simulink model "TST_DYN"  (R2020a)
settings: Solver=FixedStepAuto  StartTime=0.0  StopTime=10000  FixedStep=1  RelTol=1e-3
libraries: DYN x1
settings Model: Creator=WilTravis  LastModifiedBy=m_mam
settings DataIOCC: ReturnWorkspaceOutputs=off
settings DebuggingCC: ArithmeticOperatorsInVariantConditions=warning
settings SFSimCC: SimUseLocalCustomCode=off  CustomCodeUndefinedFunction=UseInterfaceOnly
settings RTWCC: RTWUseLocalCustomCode=off

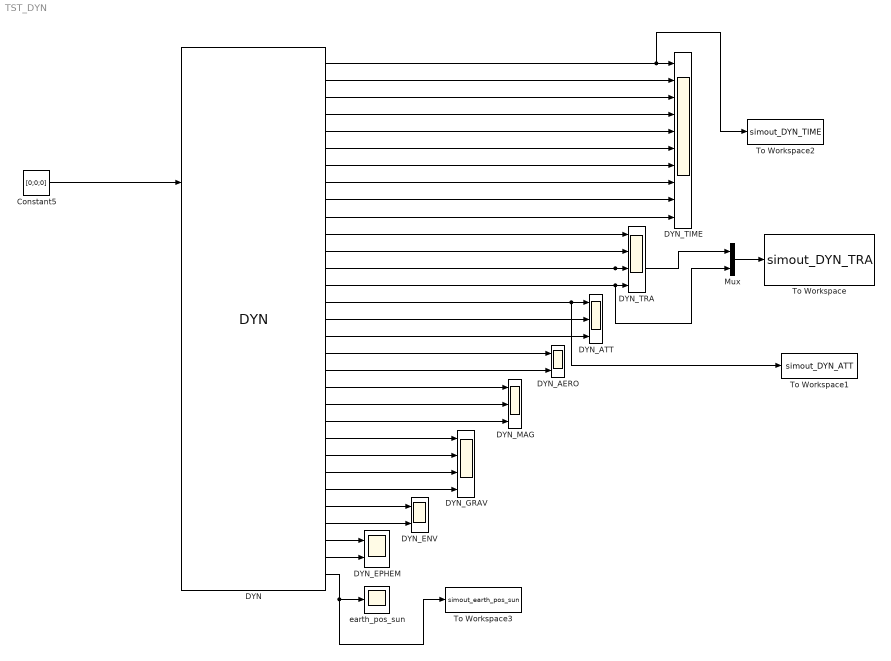
== system TST_DYN ==
  Constant5 : Constant  Value=[0;0;0]
  DYN : DYN/DYN  SystemSampleTime=-1  Latency=0  AutoFrameSizeCalculation=off
  DYN_AERO : Scope  NumInputPorts=2
  DYN_ATT : Scope  NumInputPorts=3
  DYN_ENV : Scope  NumInputPorts=2
  DYN_EPHEM : Scope  NumInputPorts=2
  DYN_GRAV : Scope  NumInputPorts=4
  DYN_MAG : Scope  NumInputPorts=3
  DYN_TIME : Scope  NumInputPorts=10
  DYN_TRA : Scope  NumInputPorts=4
  Mux : Mux  Inputs=2
  To Workspace : ToWorkspace  VariableName=simout_DYN_TRA  SaveFormat=Timeseries  SampleTime=-1
  To Workspace1 : ToWorkspace  VariableName=simout_DYN_ATT  SaveFormat=Timeseries  SampleTime=-1
  To Workspace2 : ToWorkspace  VariableName=simout_DYN_TIME  SaveFormat=Timeseries  SampleTime=-1
  To Workspace3 : ToWorkspace  VariableName=simout_earth_pos_sun  SaveFormat=Timeseries  SampleTime=-1
  earth_pos_sun : Scope
  wires:
  Constant5/1 -> DYN/1
  DYN/20 -> DYN_MAG/1
  DYN/12 -> DYN_TRA/2
  DYN/2 -> DYN_TIME/2
  DYN/28 -> DYN_ENV/2
  DYN/6 -> DYN_TIME/6
  DYN/23 -> DYN_GRAV/1
  DYN/13 -> Mux/1, DYN_TRA/3
  DYN/11 -> DYN_TRA/1
  DYN/15 -> DYN_ATT/1, To Workspace1/1
  DYN/19 -> DYN_AERO/2
  DYN/3 -> DYN_TIME/3
  DYN/24 -> DYN_GRAV/2
  DYN/4 -> DYN_TIME/4
  DYN/25 -> DYN_GRAV/3
  DYN/18 -> DYN_AERO/1
  DYN/27 -> DYN_ENV/1
  DYN/29 -> DYN_EPHEM/1
  DYN/1 -> To Workspace2/1, DYN_TIME/1
  DYN/10 -> DYN_TIME/10
  DYN/7 -> DYN_TIME/7
  DYN/8 -> DYN_TIME/8
  DYN/17 -> DYN_ATT/3
  DYN/26 -> DYN_GRAV/4
  DYN/14 -> Mux/2, DYN_TRA/4
  DYN/16 -> DYN_ATT/2
  DYN/21 -> DYN_MAG/2
  DYN/22 -> DYN_MAG/3
  DYN/9 -> DYN_TIME/9
  DYN/5 -> DYN_TIME/5
  DYN/30 -> DYN_EPHEM/2
  Mux/1 -> To Workspace/1
  DYN/31 -> To Workspace3/1, earth_pos_sun/1
